simulink model "PubIfDecisionTOS_MDL"  (R2020b)
settings: configuration reference "DspaceConfig" (kept outside this file)
PostLoadFcn:
  | if any(exist('dsrtsu_mdlpostloadfcn', 'file') ~= 0), dsrtsu_mdlpostloadfcn('Execute', bdroot); end
InitFcn:
  | , if any(exist('dsmpb_private', 'file') ~= 0), dsmpb_private('dsmpb_mdlclblib', 'Init', bdroot); end,
undefined symbols (not defined in the file or in its folder): C_TOS_ACCEgoRAxletoFbumplength_m, C_TOS_ACCTargetFront_Flag, C_TOS_AEBJAPedObjDxThre_Val, C_TOS_AEBJAPedObjDyThre_Val, C_TOS_AEBJATargetSize_Val, C_TOS_AEBJAVehObjDxThre_Val, C_TOS_AEBJAVehObjDyThre_Val, C_TOS_AEBJuncPedTargetSize_Val, C_TOS_AEBLatObjDxThre_Val, C_TOS_AEBLatPedDyThre_Val, C_TOS_AEBLatTargetSize_Val, C_TOS_AEBLongTargetInEgoFront_Flag, C_TOS_axAbsGround_Parameter, C_TOS_CameraConfirmedFlag, C_TOS_CNsubjWidth, C_TOS_CurrentLaneCoreMinWidth_Val, C_TOS_CutInProb_Val_Zero, C_TOS_CutOutProb_Val_Zero, C_TOS_D2R_Val, C_TOS_DefaultValueObjectToCenterLine_dy, C_TOS_EgoCarWidth_Val, C_TOS_EgoDxRefPoint_m, C_TOS_EgoRAxletoFbumplength_m, C_TOS_HalfWidthVehicle_Con, C_TOS_HWA_CurrentLaneFlag, C_TOS_HWA_LeftLaneFlag, C_TOS_HWA_MovingDir_Vaild, C_TOS_HWA_MovState_Vaild, C_TOS_HWA_RightLaneFlag, C_TOS_LaneLineCourseErrorFront, C_TOS_LaneLineCourseErrorRear, C_TOS_MotorbikeDefaultWidth_m, C_TOS_NumberOfEffectiveTargets, C_TOS_Obj_Age_Val, C_TOS_Objdx_Constraint_Val, C_TOS_ObjectDefaultWidth_m, C_TOS_ObjInCurrentLane_Val, C_TOS_ObjInCurrentLaneValid, C_TOS_ObjInLeftLaneValid, C_TOS_ObjInRightLaneValid, C_TOS_ObjNotInCurrentLane_Val, C_TOS_ObjNotREElementType, C_TOS_ObjPredictDis_dy_ConstantVal_Zeros, C_TOS_ObjToCenterLine_ConstantVal_Zeros, C_TOS_OFMObjIDInvilad_Val, C_TOS_PIL_LatDisCons_Val_zero, C_TOS_PIL_ObjectCutInFlag_b, C_TOS_PIL_ObjectCutOutFlag_b, C_TOS_PIL_ObjLaneProb_al_Val, C_TOS_PP_ObjFusType_FC_Confirm_b, C_TOS_PP_ObjFusType_FC_FR_Confirm_b, C_TOS_PP_ObjFusType_FR_Confirm_b, C_TOS_RE_80BoolDefault_Val, C_TOS_RE_80Single181Default_Val, C_TOS_RE_80Single255Default_Val, C_TOS_RE_80Uint8Default_Val, C_TOS_RE_D2R, C_TOS_RE_D_180_Val, C_TOS_RE_InvalidObjectID_Val, C_TOS_RE_InvalidTargetChainDir_Val ... (+142)
libraries: simulink x1650, TOS_LIB x361, canfdmsglib x14
(part 50 of 69)

== system PubIfDecisionTOS_MDL/TOS_20201112/TOS_2012080320/PP1128/AAT-AdditionalAttributes/RoadEdge/RE_2020_12_07/RoadEdge_V2/RoadEdgeElementFinalJudge/EgoRight_RoadEdgeElementsFinalJudge/Dy_Filter/If Action Subsystem ==
  Object_Dy : Inport
  Action Port : ActionPort  ActionPortLabel=if(u1|u2)
  Object_DyFilter : Outport
  wires:
  Object_Dy/1 -> Object_DyFilter/1

== system PubIfDecisionTOS_MDL/TOS_20201112/TOS_2012080320/PP1128/AAT-AdditionalAttributes/RoadEdge/RE_2020_12_07/RoadEdge_V2/RoadEdgeElementFinalJudge/EgoRight_RoadEdgeElementsFinalJudge/Dy_Filter/Subsystem ==
  Object_Dy : Inport
  Object_Dy_K1 : Inport  Port=2
  Action Port : ActionPort  ActionPortLabel=else
  Abs : Abs
  Add : Sum  Inputs=+-
  Add1 : Sum
  Constant : Constant  Value=0.2  OutDataTypeStr=single
  Gain : Gain  Gain=0.5
  Relational Operator : RelationalOperator  Operator=<  OutDataTypeStr=boolean  RndMeth=Simplest
  Switch : Switch  Criteria=u2 ~= 0
  Object_DyFilter : Outport
  wires:
  Constant/1 -> Relational Operator/2
  Object_Dy/1 -> Switch/1, Add/1
  Gain/1 -> Add1/1
  Object_Dy_K1/1 -> Add1/2, Add/2
  Abs/1 -> Relational Operator/1
  Add/1 -> Gain/1, Abs/1
  Relational Operator/1 -> Switch/2
  Add1/1 -> Switch/3
  Switch/1 -> Object_DyFilter/1

== system PubIfDecisionTOS_MDL/TOS_20201112/TOS_2012080320/PP1128/AAT-AdditionalAttributes/RoadEdge/RE_2020_12_07/RoadEdge_V2/SelectStationaryObjects/SelectStationaryObject/RE_StationaryObjectsSortCond/RE_Object_DxDy ==
  Object_Dx : Inport
  Object_Dy : Inport  Port=2
  Abs : Abs
  Compare To Constant : simulink/Logic and Bit Operations/Compare To Constant  relop=<=  const=P_TOS_RE_TargetDxMaxVal_m  OutDataTypeStr=boolean
      settings: AttributesFormatString=%<const> = 200
  Compare To Constant1 : simulink/Logic and Bit Operations/Compare To Constant  relop=>=  const=P_TOS_RE_TargetDxMinVal_m  OutDataTypeStr=boolean
      settings: AttributesFormatString=%<const> = 0
  Compare To Constant2 : simulink/Logic and Bit Operations/Compare To Constant  relop=<=  const=P_TOS_RE_TargetDyMaxVal_m  OutDataTypeStr=boolean
      settings: AttributesFormatString=%<const> = 20
  Compare To Constant3 : simulink/Logic and Bit Operations/Compare To Constant  relop=>  const=P_TOS_RE_TargetDyMinVal_m  OutDataTypeStr=boolean
      settings: AttributesFormatString=%<const> = 0.5
  Logical Operator1 : Logic  AllPortsSameDT=off  OutDataTypeStr=boolean
  Logical Operator2 : Logic  AllPortsSameDT=off  OutDataTypeStr=boolean
  Logical Operator3 : Logic  AllPortsSameDT=off  OutDataTypeStr=boolean
  RE_Object_DxDy : Outport
  wires:
  Logical Operator1/1 -> RE_Object_DxDy/1
  Object_Dx/1 -> Compare To Constant1/1, Compare To Constant/1
  Compare To Constant/1 -> Logical Operator2/1
  Compare To Constant1/1 -> Logical Operator2/2
  Logical Operator2/1 -> Logical Operator1/1
  Object_Dy/1 -> Abs/1
  Abs/1 -> Compare To Constant3/1, Compare To Constant2/1
  Compare To Constant2/1 -> Logical Operator3/1
  Compare To Constant3/1 -> Logical Operator3/2
  Logical Operator3/1 -> Logical Operator1/2

== system PubIfDecisionTOS_MDL/TOS_20201112/TOS_2012080320/PP1128/AAT-AdditionalAttributes/RoadEdge/RE_2020_12_07/RoadEdge_V2/SelectStationaryObjects/SelectStationaryObject/RE_StationaryObjectsSortCond/RE_Object_DxDyStd ==
  Object_DxStd : Inport
  Object_DyStd : Inport  Port=2
  Compare To Constant : simulink/Logic and Bit Operations/Compare To Constant  relop=<=  const=P_TOS_RE_TargetDxStdMaxVal  OutDataTypeStr=boolean
      settings: AttributesFormatString=%<const> = 12.5
  Compare To Constant2 : simulink/Logic and Bit Operations/Compare To Constant  relop=<=  const=P_TOS_RE_TargetDyStdMaxVal  OutDataTypeStr=boolean
      settings: AttributesFormatString=%<const> = 12.5
  Logical Operator1 : Logic  AllPortsSameDT=off  OutDataTypeStr=boolean
  RE_Object_DxDyStd : Outport
  wires:
  Compare To Constant2/1 -> Logical Operator1/2
  Object_DyStd/1 -> Compare To Constant2/1
  Compare To Constant/1 -> Logical Operator1/1
  Object_DxStd/1 -> Compare To Constant/1
  Logical Operator1/1 -> RE_Object_DxDyStd/1

== system PubIfDecisionTOS_MDL/TOS_20201112/TOS_2012080320/PP1128/AAT-AdditionalAttributes/RoadEdge/RE_2020_12_07/RoadEdge_V2/SelectStationaryObjects/SelectStationaryObject/RE_StationaryObjectsSortCond/RE_Object_FusType ==
  Object_FusType : Inport
  Data Type Conversion : DataTypeConversion  OutDataTypeStr=Enum: OFM_OBJ_FUSTYPE
  Enumerated Constant63 : simulink/Sources/Enumerated Constant  OutDataTypeStr=Enum: OFM_OBJ_FUSTYPE  Value=OFM_OBJ_FUSTYPE.FR  SampleTime=inf
      settings: AttributesFormatString=OFM_OBJ_FUSTYPE.FR = 2
  Enumerated Constant65 : simulink/Sources/Enumerated Constant  OutDataTypeStr=Enum: OFM_OBJ_FUSTYPE  Value=OFM_OBJ_FUSTYPE.FR_CL  SampleTime=inf
      settings: AttributesFormatString=OFM_OBJ_FUSTYPE.FR_CL = 6
  Enumerated Constant67 : simulink/Sources/Enumerated Constant  OutDataTypeStr=Enum: OFM_OBJ_FUSTYPE  Value=OFM_OBJ_FUSTYPE.FR_CR  SampleTime=inf
      settings: AttributesFormatString=OFM_OBJ_FUSTYPE.FR_CR = 10
  Enumerated Constant69 : simulink/Sources/Enumerated Constant  OutDataTypeStr=Enum: OFM_OBJ_FUSTYPE  Value=OFM_OBJ_FUSTYPE.FR_CL_CR  SampleTime=inf
      settings: AttributesFormatString=OFM_OBJ_FUSTYPE.FR_CL_CR = 14
  Enumerated Constant71 : simulink/Sources/Enumerated Constant  OutDataTypeStr=Enum: OFM_OBJ_FUSTYPE  Value=OFM_OBJ_FUSTYPE.FR_BL  SampleTime=inf
      settings: AttributesFormatString=OFM_OBJ_FUSTYPE.FR_BL = 18
  Enumerated Constant73 : simulink/Sources/Enumerated Constant  OutDataTypeStr=Enum: OFM_OBJ_FUSTYPE  Value=OFM_OBJ_FUSTYPE.FR_CL_BL  SampleTime=inf
      settings: AttributesFormatString=OFM_OBJ_FUSTYPE.FR_CL_BL = 22
  Enumerated Constant75 : simulink/Sources/Enumerated Constant  OutDataTypeStr=Enum: OFM_OBJ_FUSTYPE  Value=OFM_OBJ_FUSTYPE.FR_CR_BL  SampleTime=inf
      settings: AttributesFormatString=OFM_OBJ_FUSTYPE.FR_CR_BL = 26
  Enumerated Constant77 : simulink/Sources/Enumerated Constant  OutDataTypeStr=Enum: OFM_OBJ_FUSTYPE  Value=OFM_OBJ_FUSTYPE.FR_CL_CR_BL  SampleTime=inf
      settings: AttributesFormatString=OFM_OBJ_FUSTYPE.FR_CL_CR_BL = 30
  Enumerated Constant79 : simulink/Sources/Enumerated Constant  OutDataTypeStr=Enum: OFM_OBJ_FUSTYPE  Value=OFM_OBJ_FUSTYPE.FR_BR  SampleTime=inf
      settings: AttributesFormatString=OFM_OBJ_FUSTYPE.FR_BR = 34
  Enumerated Constant81 : simulink/Sources/Enumerated Constant  OutDataTypeStr=Enum: OFM_OBJ_FUSTYPE  Value=OFM_OBJ_FUSTYPE.FR_CL_BR  SampleTime=inf
      settings: AttributesFormatString=OFM_OBJ_FUSTYPE.FR_CL_BR = 38
  Enumerated Constant83 : simulink/Sources/Enumerated Constant  OutDataTypeStr=Enum: OFM_OBJ_FUSTYPE  Value=OFM_OBJ_FUSTYPE.FR_CR_BR  SampleTime=inf
      settings: AttributesFormatString=OFM_OBJ_FUSTYPE.FR_CR_BR = 42
  Enumerated Constant85 : simulink/Sources/Enumerated Constant  OutDataTypeStr=Enum: OFM_OBJ_FUSTYPE  Value=OFM_OBJ_FUSTYPE.FR_CL_CR_BR  SampleTime=inf
      settings: AttributesFormatString=OFM_OBJ_FUSTYPE.FR_CL_CR_BR = 46
  Enumerated Constant87 : simulink/Sources/Enumerated Constant  OutDataTypeStr=Enum: OFM_OBJ_FUSTYPE  Value=OFM_OBJ_FUSTYPE.FR_BL_BR  SampleTime=inf
      settings: AttributesFormatString=OFM_OBJ_FUSTYPE.FR_BL_BR = 50
  Enumerated Constant89 : simulink/Sources/Enumerated Constant  OutDataTypeStr=Enum: OFM_OBJ_FUSTYPE  Value=OFM_OBJ_FUSTYPE.FR_CL_BL_BR  SampleTime=inf
      settings: AttributesFormatString=OFM_OBJ_FUSTYPE.FR_CL_BL_BR = 54
  Enumerated Constant91 : simulink/Sources/Enumerated Constant  OutDataTypeStr=Enum: OFM_OBJ_FUSTYPE  Value=OFM_OBJ_FUSTYPE.FR_CR_BL_BR  SampleTime=inf
      settings: AttributesFormatString=OFM_OBJ_FUSTYPE.FR_CR_BL_BR = 58
  Enumerated Constant93 : simulink/Sources/Enumerated Constant  OutDataTypeStr=Enum: OFM_OBJ_FUSTYPE  Value=OFM_OBJ_FUSTYPE.FR_CL_CR_BL_BR  SampleTime=inf
      settings: AttributesFormatString=OFM_OBJ_FUSTYPE.FR_CL_CR_BL_BR = 62
  Logical Operator15 : Logic  Operator=OR  Inputs=16  AllPortsSameDT=off  OutDataTypeStr=boolean
  Relational Operator{16,20,22,24,26,28,30,32,34,36,38,40,42,44,46,48} (16 alike) : RelationalOperator  Operator===  OutDataTypeStr=boolean  RndMeth=Nearest
  RE_Object_FR_Other : Outport
  wires:
  Logical Operator15/1 -> RE_Object_FR_Other/1
  Enumerated Constant63/1 -> Relational Operator16/2
  Enumerated Constant65/1 -> Relational Operator20/2
  Enumerated Constant69/1 -> Relational Operator24/2
  Enumerated Constant67/1 -> Relational Operator22/2
  Enumerated Constant75/1 -> Relational Operator30/2
  Enumerated Constant77/1 -> Relational Operator32/2
  Enumerated Constant73/1 -> Relational Operator28/2
  Enumerated Constant71/1 -> Relational Operator26/2
  Enumerated Constant87/1 -> Relational Operator42/2
  Enumerated Constant89/1 -> Relational Operator44/2
  Enumerated Constant93/1 -> Relational Operator48/2
  Enumerated Constant91/1 -> Relational Operator46/2
  Object_FusType/1 -> Data Type Conversion/1
  Enumerated Constant83/1 -> Relational Operator38/2
  Enumerated Constant85/1 -> Relational Operator40/2
  Enumerated Constant81/1 -> Relational Operator36/2
  Enumerated Constant79/1 -> Relational Operator34/2
  Relational Operator16/1 -> Logical Operator15/1
  Relational Operator48/1 -> Logical Operator15/16
  Data Type Conversion/1 -> Relational Operator20/1, Relational Operator22/1, Relational Operator24/1, Relational Operator26/1, Relational Operator28/1, Relational Operator30/1, Relational Operator32/1, Relational Operator34/1, Relational Operator36/1, Relational Operator38/1, Relational Operator40/1, Relational Operator42/1, Relational Operator44/1, Relational Operator46/1, Relational Operator48/1, Relational Operator16/1
  Relational Operator20/1 -> Logical Operator15/2
  Relational Operator22/1 -> Logical Operator15/3
  Relational Operator24/1 -> Logical Operator15/4
  Relational Operator26/1 -> Logical Operator15/5
  Relational Operator28/1 -> Logical Operator15/6
  Relational Operator30/1 -> Logical Operator15/7
  Relational Operator32/1 -> Logical Operator15/8
  Relational Operator34/1 -> Logical Operator15/9
  Relational Operator36/1 -> Logical Operator15/10
  Relational Operator38/1 -> Logical Operator15/11
  Relational Operator40/1 -> Logical Operator15/12
  Relational Operator42/1 -> Logical Operator15/13
  Relational Operator44/1 -> Logical Operator15/14
  Relational Operator46/1 -> Logical Operator15/15

== system PubIfDecisionTOS_MDL/TOS_20201112/TOS_2012080320/PP1128/AAT-AdditionalAttributes/RoadEdge/RE_2020_12_07/RoadEdge_V2/SelectStationaryObjects/SelectStationaryObject/RE_StationaryObjectsSortCond/RE_Object_MovingState ==
  Object_MovingState : Inport
  Compare To Constant : simulink/Logic and Bit Operations/Compare To Constant  relop===  const=OFM_OBJ_MOVINGSTATE_E.STATIONARY  OutDataTypeStr=boolean
      settings: AttributesFormatString=%<const>
  Data Type Conversion1 : DataTypeConversion  OutDataTypeStr=Enum: OFM_OBJ_MOVINGSTATE_E
  RE_Object_Stationary : Outport
  wires:
  Data Type Conversion1/1 -> Compare To Constant/1
  Object_MovingState/1 -> Data Type Conversion1/1
  Compare To Constant/1 -> RE_Object_Stationary/1

== system PubIfDecisionTOS_MDL/TOS_20201112/TOS_2012080320/PP1128/AAT-AdditionalAttributes/RoadEdge/RE_2020_12_07/RoadEdge_V2/SelectStationaryObjects/SelectStationaryObject/RE_StationaryObjectsSortCond/Subsystem ==
  Object_ExistProb : Inport
  Object_ExistProb_K1 : Inport  Port=2
  Compare To Constant : simulink/Logic and Bit Operations/Compare To Constant  relop=>=  const=P_TOS_RE_ExistProbThre_val  OutDataTypeStr=boolean
      settings: AttributesFormatString="%<const>  = 0.4"
  Compare To Constant1 : simulink/Logic and Bit Operations/Compare To Constant  relop=>=  const=P_TOS_RE_ExistProbThre_val  OutDataTypeStr=boolean
      settings: AttributesFormatString="%<const>  = 0.4"
  Constant : Constant  Value=P_TOS_RE_stateProlongationTime  OutDataTypeStr=single
      settings: AttributesFormatString=%<Value> = 0.2
  Constant1 : Constant  Value=P_TOS_RE_Ts  OutDataTypeStr=single
      settings: AttributesFormatString=%<Value> = 0.05
  StateDelayAbortion : Stateflow chart  TreatAsAtomicUnit=on
  Terminator : Terminator
  RE_Object_ExistProb : Outport
  wires:
  Object_ExistProb/1 -> Compare To Constant/1
  Compare To Constant/1 -> StateDelayAbortion/1(state)
  StateDelayAbortion/2(stateOut) -> RE_Object_ExistProb/1
  StateDelayAbortion/1(timeSinceLastState) -> Terminator/1
  Object_ExistProb_K1/1 -> Compare To Constant1/1
  Compare To Constant1/1 -> StateDelayAbortion/2(stateK1)
  Constant/1 -> StateDelayAbortion/3(stateProlongationTime)
  Constant1/1 -> StateDelayAbortion/4(Ts)

== system PubIfDecisionTOS_MDL/TOS_20201112/TOS_2012080320/PP1128/AAT-AdditionalAttributes/RoadEdge/RE_2020_12_07/RoadEdge_V2/TargetChain/EgoLeftTargetChainDirection/Dy_Filter/If Action Subsystem ==
  Object_Dy : Inport
  Action Port : ActionPort  ActionPortLabel=if(u1|u2)
  Object_DyFilter : Outport
  wires:
  Object_Dy/1 -> Object_DyFilter/1

== system PubIfDecisionTOS_MDL/TOS_20201112/TOS_2012080320/PP1128/AAT-AdditionalAttributes/RoadEdge/RE_2020_12_07/RoadEdge_V2/TargetChain/EgoLeftTargetChainDirection/Dy_Filter/Subsystem ==
  Object_Dy : Inport
  Object_Dy_K1 : Inport  Port=2
  Action Port : ActionPort  ActionPortLabel=else
  Abs : Abs
  Add : Sum  Inputs=+-
  Add1 : Sum
  Constant : Constant  Value=0.2  OutDataTypeStr=single
  Gain : Gain  Gain=0.5
  Relational Operator : RelationalOperator  Operator=<  OutDataTypeStr=boolean  RndMeth=Simplest
  Switch : Switch  Criteria=u2 ~= 0
  Object_DyFilter : Outport
  wires:
  Constant/1 -> Relational Operator/2
  Object_Dy/1 -> Switch/1, Add/1
  Gain/1 -> Add1/1
  Object_Dy_K1/1 -> Add1/2, Add/2
  Abs/1 -> Relational Operator/1
  Add/1 -> Gain/1, Abs/1
  Relational Operator/1 -> Switch/2
  Add1/1 -> Switch/3
  Switch/1 -> Object_DyFilter/1

== system PubIfDecisionTOS_MDL/TOS_20201112/TOS_2012080320/PP1128/AAT-AdditionalAttributes/RoadEdge/RE_2020_12_07/RoadEdge_V2/TargetChain/EgoRightTargetChainDirection/Dy_Filter/If Action Subsystem ==
  Object_Dy : Inport
  Action Port : ActionPort  ActionPortLabel=if(u1|u2)
  Object_DyFilter : Outport
  wires:
  Object_Dy/1 -> Object_DyFilter/1

== system PubIfDecisionTOS_MDL/TOS_20201112/TOS_2012080320/PP1128/AAT-AdditionalAttributes/RoadEdge/RE_2020_12_07/RoadEdge_V2/TargetChain/EgoRightTargetChainDirection/Dy_Filter/Subsystem ==
  Object_Dy : Inport
  Object_Dy_K1 : Inport  Port=2
  Action Port : ActionPort  ActionPortLabel=else
  Abs : Abs
  Add : Sum  Inputs=+-
  Add1 : Sum
  Constant : Constant  Value=0.2  OutDataTypeStr=single
  Gain : Gain  Gain=0.5
  Relational Operator : RelationalOperator  Operator=<  OutDataTypeStr=boolean  RndMeth=Simplest
  Switch : Switch  Criteria=u2 ~= 0
  Object_DyFilter : Outport
  wires:
  Constant/1 -> Relational Operator/2
  Object_Dy/1 -> Switch/1, Add/1
  Gain/1 -> Add1/1
  Object_Dy_K1/1 -> Add1/2, Add/2
  Abs/1 -> Relational Operator/1
  Add/1 -> Gain/1, Abs/1
  Relational Operator/1 -> Switch/2
  Add1/1 -> Switch/3
  Switch/1 -> Object_DyFilter/1

== system PubIfDecisionTOS_MDL/TOS_20201112/TOS_2012080320/TOS/ACC/TOS_ACCCurrentLane/ACC_CurrentLane_Target/TOS_ACC_P0/ACC_P0_Targe/ACC_P0_Targe/TOS_ACC_DyConfirm/OverLapConfirm ==
  note: 弯道小于1000m,使用overlap
  note: R = 1200m
  DyConfirm_Sig : Inport
  Abs{,1..3} (4 alike) : Abs
  Add : Sum
  Bus Creator{1..4} (4 alike) : BusCreator  Inputs=2
  Bus Selector : BusSelector  OutputSignals=PositionFlag,Line_pC2
  Bus Selector1 : BusSelector  OutputSignals=PositionFlag,Line_pC2
  Bus Selector2 : BusSelector  OutputSignals=LM_LR_Line04_pC0,LM_RL_Line04_pC0
  Bus Selector3 : BusSelector  OutputSignals=PositionFlag,Line_pC2
  Bus Selector4 : BusSelector  OutputSignals=LM_LR_Line04_pC2,Object_DX,LM_LR_Line04_dDisStart,LM_LR_Line04_dDisEnd,LM_LR_Line04_fCamValid
  Bus Selector5 : BusSelector  OutputSignals=LM_LR_Line05_pC2,Object_DX,LM_LR_Line05_dDisStart,LM_LR_Line05_dDisEnd,LM_LR_Line05_fCamValid
  Bus Selector8 : BusSelector  OutputSignals=LM_LR_Line06_pC2,Object_DX,LM_LR_Line06_dDisStart,LM_LR_Line06_dDisEnd,LM_LR_Line06_fCamValid
  Compare To Constant : simulink/Logic and Bit Operations/Compare To Constant  relop===  const=uint8(4)  OutDataTypeStr=boolean
  Compare To Constant1 : simulink/Logic and Bit Operations/Compare To Constant  relop=>=  const=single(0.001)  OutDataTypeStr=boolean
  Compare To Constant2 : simulink/Logic and Bit Operations/Compare To Constant  relop=<=  const=single(0.1)  OutDataTypeStr=boolean
  Compare To Constant3 : simulink/Logic and Bit Operations/Compare To Constant  relop===  const=uint8(5)  OutDataTypeStr=boolean
  Compare To Constant4 : simulink/Logic and Bit Operations/Compare To Constant  relop=>=  const=single(0.001)  OutDataTypeStr=boolean
  Compare To Constant5 : simulink/Logic and Bit Operations/Compare To Constant  relop===  const=uint8(6)  OutDataTypeStr=boolean
  Compare To Constant6 : simulink/Logic and Bit Operations/Compare To Constant  relop=>=  const=single(0.001)  OutDataTypeStr=boolean
  Constant : Constant  Value=0  OutDataTypeStr=uint8
  Constant1 : Constant  Value=4  OutDataTypeStr=uint8
  Constant2 : Constant  Value=5  OutDataTypeStr=uint8
  Constant3 : Constant  Value=6  OutDataTypeStr=uint8
  Constant4 : Constant  Value=0  OutDataTypeStr=single
  Constant5 : Constant  OutDataTypeStr=boolean
  Logical Operator1 : Logic  AllPortsSameDT=off  OutDataTypeStr=boolean
  Logical Operator10 : Logic  Inputs=3  AllPortsSameDT=off  OutDataTypeStr=boolean
  Logical Operator11 : Logic  Inputs=3  AllPortsSameDT=off  OutDataTypeStr=boolean
  Logical Operator2 : Logic  AllPortsSameDT=off  OutDataTypeStr=boolean
  Logical Operator3 : Logic  AllPortsSameDT=off  OutDataTypeStr=boolean
  Logical Operator4 : Logic  Operator=OR  Inputs=3  AllPortsSameDT=off  OutDataTypeStr=boolean
  Logical Operator5 : Logic  Operator=OR  AllPortsSameDT=off  OutDataTypeStr=boolean
  Logical Operator6 : Logic  Operator=OR  AllPortsSameDT=off  OutDataTypeStr=boolean
  Logical Operator7 : Logic  Operator=OR  AllPortsSameDT=off  OutDataTypeStr=boolean
  Logical Operator9 : Logic  Inputs=3  AllPortsSameDT=off  OutDataTypeStr=boolean
  Relational Operator4 : RelationalOperator  Operator=>  OutDataTypeStr=boolean  RndMeth=Simplest
  Relational Operator5 : RelationalOperator  Operator=<=  OutDataTypeStr=boolean  RndMeth=Simplest
  Relational Operator6 : RelationalOperator  Operator=>  OutDataTypeStr=boolean  RndMeth=Simplest
  Relational Operator7 : RelationalOperator  Operator=<=  OutDataTypeStr=boolean  RndMeth=Simplest
  Relational Operator8 : RelationalOperator  Operator=>  OutDataTypeStr=boolean  RndMeth=Simplest
  Relational Operator9 : RelationalOperator  Operator=<=  OutDataTypeStr=boolean  RndMeth=Simplest
  Signal Copy : SignalConversion  OverrideOpt=off
  Signal Copy1 : SignalConversion  OverrideOpt=off
  Signal Copy2 : SignalConversion  OverrideOpt=off
  Switch3 : Switch  Criteria=u2 > Threshold  OutDataTypeStr=single
  Switch4 : Switch  Criteria=u2 > Threshold  OutDataTypeStr=single
  Switch5 : Switch  Criteria=u2 > Threshold  OutDataTypeStr=single
  Terminator : Terminator
  TOS_ACC_OverlapRatio : Outport
  wires:
  Abs3/1 -> Compare To Constant2/1
  Add/1 -> Abs3/1
  Logical Operator7/1 -> Logical Operator11/3
  [C0_Confirm] -> Logical Operator7/2
  Logical Operator6/1 -> Logical Operator10/3
  [C0_Confirm] -> Logical Operator6/2
  Logical Operator5/1 -> Logical Operator9/3
  [C0_Confirm] -> Logical Operator5/2
  Compare To Constant2/1 -> Terminator/1
  Bus Selector2/2 -> Add/2  "<LM_RL_Line04_pC0>"
  Bus Selector2/1 -> Add/1  "<LM_LR_Line04_pC0>"
  Abs2/1 -> Compare To Constant6/1
  Abs1/1 -> Compare To Constant4/1
  Abs/1 -> Compare To Constant1/1
  Logical Operator4/1 -> TOS_ACC_OverlapRatio/1
  Logical Operator3/1 -> Logical Operator4/3
  Logical Operator2/1 -> Logical Operator4/2
  Bus Selector3/2 -> Abs2/1  "<Line_pC2>"
  Bus Selector3/1 -> Compare To Constant5/1  "<PositionFlag>"
  Switch3/1 -> Bus Selector/1, Bus Selector1/1, Bus Selector3/1
  Compare To Constant5/1 -> Logical Operator3/1
  Compare To Constant6/1 -> Logical Operator3/2
  Compare To Constant4/1 -> Logical Operator2/2
  Compare To Constant3/1 -> Logical Operator2/1
  Bus Selector1/1 -> Compare To Constant3/1  "<PositionFlag>"
  Bus Selector1/2 -> Abs1/1  "<Line_pC2>"
  Logical Operator1/1 -> Logical Operator4/1
  Compare To Constant1/1 -> Logical Operator1/2
  DyConfirm_Sig/1 -> Bus Selector2/1, Bus Selector4/1, Bus Selector5/1, Bus Selector8/1
  Compare To Constant/1 -> Logical Operator1/1
  Bus Selector/2 -> Abs/1  "<Line_pC2>"
  Bus Selector/1 -> Compare To Constant/1  "<PositionFlag>"
  Constant4/1 -> Bus Creator4/2  "Line_pC2"
  Bus Creator3/1 -> Switch5/1
  Signal Copy2/1 -> Bus Creator3/2  "Line_pC2"
  Bus Selector4/1 -> Signal Copy/1  "<LM_LR_Line04_pC2>"
  Logical Operator9/1 -> Switch3/2
  Bus Selector5/1 -> Signal Copy1/1  "<LM_LR_Line05_pC2>"
  Constant/1 -> Bus Creator4/1  "PositionFlag"
  Signal Copy1/1 -> Bus Creator2/2  "Line_pC2"
  Constant3/1 -> Bus Creator3/1  "PositionFlag"
  Constant2/1 -> Bus Creator2/1  "PositionFlag"
  Bus Selector4/4 -> Relational Operator5/2  "<LM_LR_Line04_dDisEnd>"
  Bus Creator4/1 -> Switch5/3
  Relational Operator7/1 -> Logical Operator10/2
  Relational Operator6/1 -> Logical Operator10/1
  Constant1/1 -> Bus Creator1/1  "PositionFlag"
  Relational Operator4/1 -> Logical Operator9/1
  Bus Creator2/1 -> Switch4/1
  Bus Selector5/5 -> Logical Operator6/1  "<LM_LR_Line05_fCamValid>"
  Switch5/1 -> Switch4/3
  Bus Selector8/5 -> Logical Operator7/1  "<LM_LR_Line06_fCamValid>"
  Bus Selector5/2 -> Relational Operator7/1, Relational Operator6/1  "<Object_DX>"
  Bus Selector5/3 -> Relational Operator6/2  "<LM_LR_Line05_dDisStart>"
  Logical Operator11/1 -> Switch5/2
  Bus Creator1/1 -> Switch3/1
  Bus Selector8/4 -> Relational Operator9/2  "<LM_LR_Line06_dDisEnd>"
  Switch4/1 -> Switch3/3
  Relational Operator9/1 -> Logical Operator11/2
  Bus Selector8/1 -> Signal Copy2/1  "<LM_LR_Line06_pC2>"
  Bus Selector8/3 -> Relational Operator8/2  "<LM_LR_Line06_dDisStart>"
  Signal Copy/1 -> Bus Creator1/2  "Line_pC2"
  Relational Operator5/1 -> Logical Operator9/2
  Relational Operator8/1 -> Logical Operator11/1
  Bus Selector4/2 -> Relational Operator4/1, Relational Operator5/1  "<Object_DX>"
  Bus Selector5/4 -> Relational Operator7/2  "<LM_LR_Line05_dDisEnd>"
  Bus Selector4/3 -> Relational Operator4/2  "<LM_LR_Line04_dDisStart>"
  Bus Selector4/5 -> Logical Operator5/1  "<LM_LR_Line04_fCamValid>"
  Bus Selector8/2 -> Relational Operator8/1, Relational Operator9/1  "<Object_DX>"
  Logical Operator10/1 -> Switch4/2
  Constant5/1 -> [C0_Confirm]

== system PubIfDecisionTOS_MDL/TOS_20201112/TOS_2012080320/TOS/ACC/TOS_ACCCurrentLane/ACC_CurrentLane_Target/TOS_ACC_P0/ACC_P0_Targe/ACC_P0_Targe/TOS_ACC_DyConfirm/OverLapConfirm_V0318（） ==
  note: R = 1200m
  DyConfirm_Sig : Inport
  Abs{,1..3} (4 alike) : Abs
  Add : Sum
  Bus Creator{1..4} (4 alike) : BusCreator  Inputs=2
  Bus Selector : BusSelector  OutputSignals=PositionFlag,Line_pC2
  Bus Selector1 : BusSelector  OutputSignals=PositionFlag,Line_pC2
  Bus Selector2 : BusSelector  OutputSignals=LM_LR_Line04_pC0,LM_RL_Line04_pC0
  Bus Selector3 : BusSelector  OutputSignals=PositionFlag,Line_pC2
  Bus Selector4 : BusSelector  OutputSignals=LM_LR_Line04_pC2,Object_DX,LM_LR_Line04_dDisStart,LM_LR_Line04_dDisEnd,LM_LR_Line04_fCamValid
  Bus Selector5 : BusSelector  OutputSignals=LM_LR_Line05_pC2,Object_DX,LM_LR_Line05_dDisStart,LM_LR_Line05_dDisEnd,LM_LR_Line05_fCamValid
  Bus Selector8 : BusSelector  OutputSignals=LM_LR_Line06_pC2,Object_DX,LM_LR_Line06_dDisStart,LM_LR_Line06_dDisEnd,LM_LR_Line06_fCamValid
  Compare To Constant : simulink/Logic and Bit Operations/Compare To Constant  relop===  const=uint8(4)  OutDataTypeStr=boolean
  Compare To Constant1 : simulink/Logic and Bit Operations/Compare To Constant  relop=>=  const=single(0.001)  OutDataTypeStr=boolean
  Compare To Constant2 : simulink/Logic and Bit Operations/Compare To Constant  relop=<=  const=single(0.1)  OutDataTypeStr=boolean
  Compare To Constant3 : simulink/Logic and Bit Operations/Compare To Constant  relop===  const=uint8(5)  OutDataTypeStr=boolean
  Compare To Constant4 : simulink/Logic and Bit Operations/Compare To Constant  relop=>=  const=single(0.001)  OutDataTypeStr=boolean
  Compare To Constant5 : simulink/Logic and Bit Operations/Compare To Constant  relop===  const=uint8(6)  OutDataTypeStr=boolean
  Compare To Constant6 : simulink/Logic and Bit Operations/Compare To Constant  relop=>=  const=single(0.001)  OutDataTypeStr=boolean
  Constant : Constant  Value=0  OutDataTypeStr=uint8
  Constant1 : Constant  Value=4  OutDataTypeStr=uint8
  Constant2 : Constant  Value=5  OutDataTypeStr=uint8
  Constant3 : Constant  Value=6  OutDataTypeStr=uint8
  Constant4 : Constant  Value=0  OutDataTypeStr=single
  Logical Operator1 : Logic  AllPortsSameDT=off  OutDataTypeStr=boolean
  Logical Operator10 : Logic  Inputs=3  AllPortsSameDT=off  OutDataTypeStr=boolean
  Logical Operator11 : Logic  Inputs=3  AllPortsSameDT=off  OutDataTypeStr=boolean
  Logical Operator2 : Logic  AllPortsSameDT=off  OutDataTypeStr=boolean
  Logical Operator3 : Logic  AllPortsSameDT=off  OutDataTypeStr=boolean
  Logical Operator4 : Logic  Operator=OR  Inputs=3  AllPortsSameDT=off  OutDataTypeStr=boolean
  Logical Operator5 : Logic  Operator=OR  AllPortsSameDT=off  OutDataTypeStr=boolean
  Logical Operator6 : Logic  Operator=OR  AllPortsSameDT=off  OutDataTypeStr=boolean
  Logical Operator7 : Logic  Operator=OR  AllPortsSameDT=off  OutDataTypeStr=boolean
  Logical Operator9 : Logic  Inputs=3  AllPortsSameDT=off  OutDataTypeStr=boolean
  Relational Operator4 : RelationalOperator  Operator=>  OutDataTypeStr=boolean  RndMeth=Simplest
  Relational Operator5 : RelationalOperator  Operator=<=  OutDataTypeStr=boolean  RndMeth=Simplest
  Relational Operator6 : RelationalOperator  Operator=>  OutDataTypeStr=boolean  RndMeth=Simplest
  Relational Operator7 : RelationalOperator  Operator=<=  OutDataTypeStr=boolean  RndMeth=Simplest
  Relational Operator8 : RelationalOperator  Operator=>  OutDataTypeStr=boolean  RndMeth=Simplest
  Relational Operator9 : RelationalOperator  Operator=<=  OutDataTypeStr=boolean  RndMeth=Simplest
  Signal Copy : SignalConversion  OverrideOpt=off
  Signal Copy1 : SignalConversion  OverrideOpt=off
  Signal Copy2 : SignalConversion  OverrideOpt=off
  Switch3 : Switch  Criteria=u2 > Threshold  OutDataTypeStr=single
  Switch4 : Switch  Criteria=u2 > Threshold  OutDataTypeStr=single
  Switch5 : Switch  Criteria=u2 > Threshold  OutDataTypeStr=single
  TOS_ACC_OverlapRatio : Outport
  wires:
  Logical Operator10/1 -> Switch4/2
  Bus Selector8/2 -> Relational Operator9/1, Relational Operator8/1  "<Object_DX>"
  Bus Selector4/5 -> Logical Operator5/1  "<LM_LR_Line04_fCamValid>"
  Bus Selector4/3 -> Relational Operator4/2  "<LM_LR_Line04_dDisStart>"
  Bus Selector5/4 -> Relational Operator7/2  "<LM_LR_Line05_dDisEnd>"
  Bus Selector4/2 -> Relational Operator5/1, Relational Operator4/1  "<Object_DX>"
  Relational Operator8/1 -> Logical Operator11/1
  Relational Operator5/1 -> Logical Operator9/2
  Signal Copy/1 -> Bus Creator1/2  "Line_pC2"
  Bus Selector8/3 -> Relational Operator8/2  "<LM_LR_Line06_dDisStart>"
  Bus Selector8/1 -> Signal Copy2/1  "<LM_LR_Line06_pC2>"
  Relational Operator9/1 -> Logical Operator11/2
  Switch4/1 -> Switch3/3
  Bus Selector8/4 -> Relational Operator9/2  "<LM_LR_Line06_dDisEnd>"
  Bus Creator1/1 -> Switch3/1
  Logical Operator11/1 -> Switch5/2
  Bus Selector5/3 -> Relational Operator6/2  "<LM_LR_Line05_dDisStart>"
  Bus Selector5/2 -> Relational Operator6/1, Relational Operator7/1  "<Object_DX>"
  Bus Selector8/5 -> Logical Operator7/1  "<LM_LR_Line06_fCamValid>"
  Switch5/1 -> Switch4/3
  Bus Selector5/5 -> Logical Operator6/1  "<LM_LR_Line05_fCamValid>"
  Bus Creator2/1 -> Switch4/1
  Relational Operator4/1 -> Logical Operator9/1
  Constant1/1 -> Bus Creator1/1  "PositionFlag"
  Relational Operator6/1 -> Logical Operator10/1
  Relational Operator7/1 -> Logical Operator10/2
  Bus Creator4/1 -> Switch5/3
  Bus Selector4/4 -> Relational Operator5/2  "<LM_LR_Line04_dDisEnd>"
  Constant2/1 -> Bus Creator2/1  "PositionFlag"
  Constant3/1 -> Bus Creator3/1  "PositionFlag"
  Signal Copy1/1 -> Bus Creator2/2  "Line_pC2"
  Constant/1 -> Bus Creator4/1  "PositionFlag"
  Bus Selector5/1 -> Signal Copy1/1  "<LM_LR_Line05_pC2>"
  Logical Operator9/1 -> Switch3/2
  Bus Selector4/1 -> Signal Copy/1  "<LM_LR_Line04_pC2>"
  Signal Copy2/1 -> Bus Creator3/2  "Line_pC2"
  Bus Creator3/1 -> Switch5/1
  Constant4/1 -> Bus Creator4/2  "Line_pC2"
  Bus Selector/1 -> Compare To Constant/1  "<PositionFlag>"
  Bus Selector/2 -> Abs/1  "<Line_pC2>"
  Compare To Constant/1 -> Logical Operator1/1
  DyConfirm_Sig/1 -> Bus Selector8/1, Bus Selector5/1, Bus Selector4/1, Bus Selector2/1
  Compare To Constant1/1 -> Logical Operator1/2
  Logical Operator1/1 -> Logical Operator4/1
  Bus Selector1/2 -> Abs1/1  "<Line_pC2>"
  Bus Selector1/1 -> Compare To Constant3/1  "<PositionFlag>"
  Compare To Constant3/1 -> Logical Operator2/1
  Compare To Constant4/1 -> Logical Operator2/2
  Compare To Constant6/1 -> Logical Operator3/2
  Compare To Constant5/1 -> Logical Operator3/1
  Switch3/1 -> Bus Selector3/1, Bus Selector1/1, Bus Selector/1
  Bus Selector3/1 -> Compare To Constant5/1  "<PositionFlag>"
  Bus Selector3/2 -> Abs2/1  "<Line_pC2>"
  Logical Operator2/1 -> Logical Operator4/2
  Logical Operator3/1 -> Logical Operator4/3
  Logical Operator4/1 -> TOS_ACC_OverlapRatio/1
  Abs/1 -> Compare To Constant1/1
  Abs1/1 -> Compare To Constant4/1
  Abs2/1 -> Compare To Constant6/1
  Bus Selector2/1 -> Add/1  "<LM_LR_Line04_pC0>"
  Bus Selector2/2 -> Add/2  "<LM_RL_Line04_pC0>"
  Compare To Constant2/1 -> [C0_Confirm]
  [C0_Confirm] -> Logical Operator5/2
  Logical Operator5/1 -> Logical Operator9/3
  [C0_Confirm] -> Logical Operator6/2
  Logical Operator6/1 -> Logical Operator10/3
  [C0_Confirm] -> Logical Operator7/2
  Logical Operator7/1 -> Logical Operator11/3
  Add/1 -> Abs3/1
  Abs3/1 -> Compare To Constant2/1

== system PubIfDecisionTOS_MDL/TOS_20201112/TOS_2012080320/TOS/ACC/TOS_ACCCurrentLane/ACC_CurrentLane_Target/TOS_ACC_P0/ACC_P0_Targe/ACC_P0_Targe/TOS_ACC_DyConfirm/TOS_ACC_DyConfirm_V3.14 ==
  Object_DY : Inport
  Object_DX : Inport  Port=2
  <Object_Type> : Inport  Port=3
  Abs{,1..3} (4 alike) : Abs
  Bus Creator : BusCreator  Inputs=3
  Bus Selector : BusSelector  OutputSignals=Object_Type
  Bus Selector1 : BusSelector  OutputSignals=Object_DY
  Bus Selector2 : BusSelector  OutputSignals=Object_DX
  Bus Selector3 : BusSelector  OutputSignals=Object_Type
  Bus Selector4 : BusSelector  OutputSignals=Object_DY
  Bus Selector5 : BusSelector  OutputSignals=Object_DX
  Compare To Constant1 : simulink/Logic and Bit Operations/Compare To Constant  relop===  const=OFM_OBJ_TYPE_E.UNKNOWN_TYPE  OutDataTypeStr=boolean
      settings: AttributesFormatString=OFM_OBJ_TYPE_E.UNKNOWN_TYPE = 1
  Compare To Constant10 : simulink/Logic and Bit Operations/Compare To Constant  relop===  const=OFM_OBJ_TYPE_E.CAR  OutDataTypeStr=boolean
      settings: AttributesFormatString=OFM_OBJ_TYPE_E.CAR = 2
  Compare To Constant2 : simulink/Logic and Bit Operations/Compare To Constant  relop===  const=OFM_OBJ_TYPE_E.MOTORBIKE  OutDataTypeStr=boolean
      settings: AttributesFormatString=OFM_OBJ_TYPE_E.MOTORBIKE = 4
  Compare To Constant3 : simulink/Logic and Bit Operations/Compare To Constant  relop===  const=OFM_OBJ_TYPE_E.PEDESTRIAN  OutDataTypeStr=boolean
      settings: AttributesFormatString=OFM_OBJ_TYPE_E.PEDESTRIAN = 6
  Compare To Constant4 : simulink/Logic and Bit Operations/Compare To Constant  relop===  const=OFM_OBJ_TYPE_E.BICYCLE  OutDataTypeStr=boolean
      settings: AttributesFormatString=OFM_OBJ_TYPE_E.BICYCLE = 5
  Compare To Constant5 : simulink/Logic and Bit Operations/Compare To Constant  relop===  const=OFM_OBJ_TYPE_E.GENERAL_OBJECT  OutDataTypeStr=boolean
      settings: AttributesFormatString=OFM_OBJ_TYPE_E.GENERAL_OBJECT = 7
  Compare To Constant6 : simulink/Logic and Bit Operations/Compare To Constant  relop===  const=OFM_OBJ_TYPE_E.ANIMAL  OutDataTypeStr=boolean
      settings: AttributesFormatString=OFM_OBJ_TYPE_E.ANIMAL = 8
  Compare To Constant7 : simulink/Logic and Bit Operations/Compare To Constant  relop===  const=OFM_OBJ_TYPE_E.INVALID  OutDataTypeStr=boolean
      settings: AttributesFormatString=OFM_OBJ_TYPE_E.INVALID = 0
  Compare To Constant8 : simulink/Logic and Bit Operations/Compare To Constant  relop===  const=OFM_OBJ_TYPE_E.TRUCK  OutDataTypeStr=boolean
      settings: AttributesFormatString=OFM_OBJ_TYPE_E.TRUCK = 3
  Data Type Conversion1 : DataTypeConversion  OutDataTypeStr=Enum: OFM_OBJ_TYPE_E
  Data Type Conversion2 : DataTypeConversion  OutDataTypeStr=Enum: OFM_OBJ_TYPE_E
  Logical Operator : Logic  AllPortsSameDT=off  OutDataTypeStr=boolean
  Logical Operator1 : Logic  Operator=OR  Inputs=7  AllPortsSameDT=off  OutDataTypeStr=boolean
  Logical Operator2 : Logic  AllPortsSameDT=off  OutDataTypeStr=boolean
  Logical Operator3 : Logic  Operator=OR  AllPortsSameDT=off  OutDataTypeStr=boolean
  Logical Operator4 : Logic  Operator=OR  AllPortsSameDT=off  OutDataTypeStr=boolean
  Relational Operator : RelationalOperator  Operator=<=  OutDataTypeStr=boolean  RndMeth=Simplest
  Relational Operator1 : RelationalOperator  Operator=<=  OutDataTypeStr=boolean  RndMeth=Simplest
  data1 : Lookup_n-D  NumberOfTableDimensions=1  BreakpointsForDimension1=[0,20,40,60,80,100,120,140]  Table=[1.5,1.5,1.45,1.45,1.4,1.4,1.4,1.4]  RndMeth=Simplest  InputSameDT=on
  data3 : Lookup_n-D  NumberOfTableDimensions=1  BreakpointsForDimension1=[0,40,45,55,60,65,70,95,115,140]  Table=[2.5,2.5,2.5,2.5,3,3,3,3,3.2,3.2]  RndMeth=Simplest  InputSameDT=on
  data4 : Lookup_n-D  NumberOfTableDimensions=1  BreakpointsForDimension1=[0,40,45,55,60,65,70,95,115,140]  Table=[1.4,1.5,1.7,1.7,2,2,2,2,2.5,2.5]  RndMeth=Simplest  InputSameDT=on
  TOS_ACC_DyConfirm : Outport
  wires:
  Object_DX/1 -> Bus Creator/2
  Object_DY/1 -> Bus Creator/1
  Relational Operator/1 -> Logical Operator/1
  Abs/1 -> data4/1
  data4/1 -> Relational Operator/2
  Abs1/1 -> Relational Operator/1
  <Object_Type>/1 -> Bus Creator/3
  Bus Selector/1 -> Data Type Conversion2/1  "<Object_Type>"
  Compare To Constant3/1 -> Logical Operator1/1
  Bus Selector2/1 -> Abs/1  "<Object_DX>"
  Bus Selector1/1 -> Abs1/1  "<Object_DY>"
  Data Type Conversion2/1 -> Compare To Constant7/1, Compare To Constant6/1, Compare To Constant5/1, Compare To Constant4/1, Compare To Constant2/1, Compare To Constant1/1, Compare To Constant3/1
  Compare To Constant1/1 -> Logical Operator1/2
  Compare To Constant2/1 -> Logical Operator1/3
  Compare To Constant4/1 -> Logical Operator1/4
  Compare To Constant5/1 -> Logical Operator1/5
  Compare To Constant6/1 -> Logical Operator1/6
  Compare To Constant7/1 -> Logical Operator1/7
  Logical Operator1/1 -> Logical Operator/2
  Logical Operator3/1 -> Logical Operator2/2
  Compare To Constant8/1 -> Logical Operator3/2
  Data Type Conversion1/1 -> Compare To Constant10/1, Compare To Constant8/1
  Bus Selector4/1 -> Abs3/1  "<Object_DY>"
  Bus Selector5/1 -> Abs2/1  "<Object_DX>"
  Compare To Constant10/1 -> Logical Operator3/1
  Bus Selector3/1 -> Data Type Conversion1/1  "<Object_Type>"
  Bus Creator/1 -> Bus Selector2/1, Bus Selector4/1, Bus Selector3/1, Bus Selector5/1, Bus Selector/1, Bus Selector1/1
  Abs3/1 -> Relational Operator1/1
  data3/1 -> Relational Operator1/2
  Abs2/1 -> data3/1
  Relational Operator1/1 -> Logical Operator2/1
  Logical Operator/1 -> Logical Operator4/1
  Logical Operator2/1 -> Logical Operator4/2
  Logical Operator4/1 -> TOS_ACC_DyConfirm/1

== system PubIfDecisionTOS_MDL/TOS_20201112/TOS_2012080320/TOS/ACC/TOS_ACCCurrentLane/ACC_CurrentLane_Target/TOS_ACC_P0/ACC_P0_Targe/ACC_P0_Targe/TOS_ACC_DyConfirm/TOS_ACC_DyConfirm_V3.15 ==
  Object_DY : Inport
  Object_DX : Inport  Port=2
  Object_Type : Inport  Port=3
  object_MovingState : Inport  Port=4
  Abs{,1..7} (8 alike) : Abs
  Bus Creator : BusCreator  Inputs=4
  Bus Selector1 : BusSelector  OutputSignals=Object_DY,Object_DX
  Bus Selector3 : BusSelector  OutputSignals=Object_DY,Object_DX,Object_Type
  Bus Selector6 : BusSelector  OutputSignals=Object_DY,Object_DX,object_MovingState
  Bus Selector7 : BusSelector  OutputSignals=Object_DY,Object_DX,Object_Type
  Compare To Constant1 : simulink/Logic and Bit Operations/Compare To Constant  relop===  const=OFM_OBJ_TYPE_E.UNKNOWN_TYPE  OutDataTypeStr=boolean
      settings: AttributesFormatString=OFM_OBJ_TYPE_E.UNKNOWN_TYPE = 1
  Compare To Constant10 : simulink/Logic and Bit Operations/Compare To Constant  relop===  const=OFM_OBJ_TYPE_E.CAR  OutDataTypeStr=boolean
      settings: AttributesFormatString=OFM_OBJ_TYPE_E.CAR = 2
  Compare To Constant11 : simulink/Logic and Bit Operations/Compare To Constant  relop===  const=OFM_OBJ_MOVINGSTATE_E.STATIONARY  OutDataTypeStr=boolean
      settings: AttributesFormatString=OFM_OBJ_MOVINGSTATE_E.UNKNOWN = 3
  Compare To Constant2 : simulink/Logic and Bit Operations/Compare To Constant  relop===  const=OFM_OBJ_TYPE_E.MOTORBIKE  OutDataTypeStr=boolean
      settings: AttributesFormatString=OFM_OBJ_TYPE_E.MOTORBIKE = 4
  Compare To Constant3 : simulink/Logic and Bit Operations/Compare To Constant  relop===  const=OFM_OBJ_TYPE_E.PEDESTRIAN  OutDataTypeStr=boolean
      settings: AttributesFormatString=OFM_OBJ_TYPE_E.PEDESTRIAN = 6
  Compare To Constant4 : simulink/Logic and Bit Operations/Compare To Constant  relop===  const=OFM_OBJ_TYPE_E.BICYCLE  OutDataTypeStr=boolean
      settings: AttributesFormatString=OFM_OBJ_TYPE_E.BICYCLE = 5
  Compare To Constant5 : simulink/Logic and Bit Operations/Compare To Constant  relop===  const=OFM_OBJ_TYPE_E.GENERAL_OBJECT  OutDataTypeStr=boolean
      settings: AttributesFormatString=OFM_OBJ_TYPE_E.GENERAL_OBJECT = 7
  Compare To Constant6 : simulink/Logic and Bit Operations/Compare To Constant  relop===  const=OFM_OBJ_TYPE_E.ANIMAL  OutDataTypeStr=boolean
      settings: AttributesFormatString=OFM_OBJ_TYPE_E.ANIMAL = 8
  Compare To Constant8 : simulink/Logic and Bit Operations/Compare To Constant  relop===  const=OFM_OBJ_TYPE_E.TRUCK  OutDataTypeStr=boolean
      settings: AttributesFormatString=OFM_OBJ_TYPE_E.TRUCK = 3
  Compare To Constant9 : simulink/Logic and Bit Operations/Compare To Constant  relop===  const=OFM_OBJ_MOVINGSTATE_E.UNKNOWN  OutDataTypeStr=boolean
      settings: AttributesFormatString=OFM_OBJ_MOVINGSTATE_E.UNKNOWN = 1
  Data Type Conversion1 : DataTypeConversion  OutDataTypeStr=Enum: OFM_OBJ_TYPE_E
  Data Type Conversion2 : DataTypeConversion  OutDataTypeStr=Enum: OFM_OBJ_TYPE_E
  Data Type Conversion3 : DataTypeConversion  OutDataTypeStr=Enum: OFM_OBJ_MOVINGSTATE_E
  Logical Operator1 : Logic  Operator=OR  Inputs=6  AllPortsSameDT=off  OutDataTypeStr=boolean
  Logical Operator3 : Logic  Operator=OR  AllPortsSameDT=off  OutDataTypeStr=boolean
  Logical Operator6 : Logic  Operator=OR  AllPortsSameDT=off  OutDataTypeStr=boolean
  Relational Operator{,1..3} (4 alike) : RelationalOperator  Operator=<=  OutDataTypeStr=boolean  RndMeth=Simplest
  Switch : Switch  Criteria=u2 > Threshold
  Switch1 : Switch  Criteria=u2 > Threshold
  Switch2 : Switch  Criteria=u2 > Threshold
  data1 : Lookup_n-D  NumberOfTableDimensions=1  BreakpointsForDimension1=[0,20,40,60,80,100,120,140]  Table=[1.5,1.5,1.45,1.45,1.4,1.4,1.4,1.4]  RndMeth=Simplest  InputSameDT=on
  data3 : Lookup_n-D  NumberOfTableDimensions=1  BreakpointsForDimension1=[0,20,40,60,80,100,120,140]  Table=[1.4,1.4,1.3,1.3,1.2,1.2,1.2,1.2]  RndMeth=Simplest  InputSameDT=on
  data4 : Lookup_n-D  NumberOfTableDimensions=1  BreakpointsForDimension1=[0,20,40,60,80,100,120,140]  Table=[1.4,1.4,1.3,1.3,1.2,1.2,1.2,1.2]  RndMeth=Simplest  InputSameDT=on
  data5 : Lookup_n-D  NumberOfTableDimensions=1  BreakpointsForDimension1=[0,20,40,60,80,100,120,140]  Table=[1.9,1.9,1.85,1.85,1.8,1.8,1.8,1.8]  RndMeth=Simplest  InputSameDT=on
  TOS_ACC_DyConfirm : Outport
  TOS_ACC_P0_P1_DyConfirm_1_ObserVale : Outport  Port=2
  TOS_ACC_P0_P1_DyConfirm_2_ObserVale : Outport  Port=3
  TOS_ACC_P0_P1_DyConfirm_3_ObserVale : Outport  Port=4
  wires:
  Switch/1 -> TOS_ACC_DyConfirm/1
  Abs2/1 -> data5/1
  data5/1 -> Relational Operator1/2
  Abs3/1 -> Relational Operator1/1
  Bus Selector7/3 -> Data Type Conversion1/1  "<Object_Type>"
  Compare To Constant10/1 -> Logical Operator3/1
  Bus Selector7/2 -> Abs2/1  "<Object_DX>"
  Bus Selector7/1 -> Abs3/1  "<Object_DY>"
  Data Type Conversion1/1 -> Compare To Constant8/1, Compare To Constant10/1
  Compare To Constant8/1 -> Logical Operator3/2
  Logical Operator1/1 -> [TOS_ACC_P0_P1_DyConfirm_3_ObserVale], Switch2/2
  Compare To Constant6/1 -> Logical Operator1/6
  Compare To Constant5/1 -> Logical Operator1/5
  Compare To Constant4/1 -> Logical Operator1/4
  Compare To Constant2/1 -> Logical Operator1/3
  Compare To Constant1/1 -> Logical Operator1/2
  Data Type Conversion2/1 -> Compare To Constant3/1, Compare To Constant6/1, Compare To Constant5/1, Compare To Constant4/1, Compare To Constant2/1, Compare To Constant1/1
  Bus Selector3/1 -> Abs1/1  "<Object_DY>"
  Bus Selector3/2 -> Abs/1  "<Object_DX>"
  Compare To Constant3/1 -> Logical Operator1/1
  Bus Selector3/3 -> Data Type Conversion2/1  "<Object_Type>"
  Object_Type/1 -> Bus Creator/3  "Object_Type"
  Abs1/1 -> Relational Operator/1
  data3/1 -> Relational Operator/2
  Abs/1 -> data3/1
  Relational Operator/1 -> Switch2/1
  Object_DY/1 -> Bus Creator/1  "Object_DY"
  Object_DX/1 -> Bus Creator/2  "Object_DX"
  Bus Creator/1 -> Bus Selector1/1, Bus Selector3/1, Bus Selector7/1, Bus Selector6/1
  Compare To Constant11/1 -> Logical Operator6/2
  Compare To Constant9/1 -> Logical Operator6/1
  object_MovingState/1 -> Bus Creator/4  "object_MovingState"
  Bus Selector6/3 -> Data Type Conversion3/1  "<object_MovingState>"
  Bus Selector6/1 -> Abs4/1  "<Object_DY>"
  Bus Selector6/2 -> Abs5/1  "<Object_DX>"
  Abs5/1 -> data1/1
  data1/1 -> Relational Operator2/2
  Abs4/1 -> Relational Operator2/1
  Logical Operator6/1 -> [TOS_ACC_P0_P1_DyConfirm_1_ObserVale], Switch/2
  Relational Operator2/1 -> Switch/1
  Logical Operator3/1 -> [TOS_ACC_P0_P1_DyConfirm_2_ObserVale], Switch1/2
  Relational Operator1/1 -> Switch1/1
  Switch1/1 -> Switch/3
  Switch2/1 -> Switch1/3
  Bus Selector1/2 -> Abs6/1  "<Object_DX>"
  Bus Selector1/1 -> Abs7/1  "<Object_DY>"
  Abs6/1 -> data4/1
  data4/1 -> Relational Operator3/2
  Abs7/1 -> Relational Operator3/1
  Relational Operator3/1 -> Switch2/3
  [TOS_ACC_P0_P1_DyConfirm_1_ObserVale] -> TOS_ACC_P0_P1_DyConfirm_1_ObserVale/1
  [TOS_ACC_P0_P1_DyConfirm_2_ObserVale] -> TOS_ACC_P0_P1_DyConfirm_2_ObserVale/1
  [TOS_ACC_P0_P1_DyConfirm_3_ObserVale] -> TOS_ACC_P0_P1_DyConfirm_3_ObserVale/1
  Data Type Conversion3/1 -> Compare To Constant11/1, Compare To Constant9/1  "object_MovingState"

== system PubIfDecisionTOS_MDL/TOS_20201112/TOS_2012080320/TOS/ACC/TOS_ACCCurrentLane/ACC_CurrentLane_Target/TOS_ACC_P0/ACC_P0_Targe/ACC_P0_Targe/TOS_ACC_FusionTypeConfirm/Subsystem1 ==
  ObjMovState : Inport
  ACC_Target_ID_K1 : Inport  Port=2
  ACC_Target_ID_K2 : Inport  Port=3
  ACC_Target_MovState_K1 : Inport  Port=4
  ACC_Target_MovState_K2 : Inport  Port=5
  ObjectID : Inport  Port=6
  TOS_ObjMovStateCfmFlow1 : Stateflow chart  TreatAsAtomicUnit=on
  TOS_ObjMovStateCfm : Outport
  wires:
  TOS_ObjMovStateCfmFlow1/1(TOS_ObjMovStateCfm) -> TOS_ObjMovStateCfm/1
  ACC_Target_ID_K1/1 -> TOS_ObjMovStateCfmFlow1/1(Target_ID_K1)
  ACC_Target_ID_K2/1 -> TOS_ObjMovStateCfmFlow1/2(Target_ID_K2)
  ACC_Target_MovState_K1/1 -> TOS_ObjMovStateCfmFlow1/3(Target_MovState_K1)
  ACC_Target_MovState_K2/1 -> TOS_ObjMovStateCfmFlow1/4(Target_MovState_K2)
  ObjMovState/1 -> TOS_ObjMovStateCfmFlow1/5(ObjMovState)
  ObjectID/1 -> TOS_ObjMovStateCfmFlow1/6(ObjectID)

== system PubIfDecisionTOS_MDL/TOS_20201112/TOS_2012080320/TOS/ACC/TOS_ACCCurrentLane/ACC_CurrentLane_Target/TOS_ACC_P0/ACC_P0_Targe/ACC_P0_Targe/TOS_ACC_FusionTypeConfirm/TOS_ACCFusionTypeAborDly ==
  ACC_TargetP0_ID_K1 : Inport
  ObjectID : Inport  Port=2
  TOS_ACCFusionType : Inport  Port=3
  If : If  IfExpression=u1
  If Action Subsystem : Subsystem  TreatAsAtomicUnit=on
  If Action Subsystem1 : Subsystem  TreatAsAtomicUnit=on
  Merge : Merge
  Relational Operator : RelationalOperator  Operator===  OutDataTypeStr=boolean  RndMeth=Simplest
  TOS_ACCFusionTypeFilt : Outport
  wires:
  If/1 -> If Action Subsystem1/Action
  TOS_ACCFusionType/1 -> If Action Subsystem1/1(TOS_ACCFusionType), If Action Subsystem/1(TOS_ACCFusionType)
  If/2 -> If Action Subsystem/Action
  ACC_TargetP0_ID_K1/1 -> Relational Operator/1
  ObjectID/1 -> Relational Operator/2
  Relational Operator/1 -> If/1
  If Action Subsystem1/1(TOS_ACCFusionTypeFilt) -> Merge/1
  If Action Subsystem/1(TOS_ACCFusionTypeFilt) -> Merge/2
  Merge/1 -> TOS_ACCFusionTypeFilt/1

== system PubIfDecisionTOS_MDL/TOS_20201112/TOS_2012080320/TOS/ACC/TOS_ACCCurrentLane/ACC_CurrentLane_Target/TOS_ACC_P0/ACC_P0_Targe/ACC_P0_Targe/TOS_ACC_ObjTypeConfirm/Subsystem ==
  ObjMovState : Inport
  ACC_Target_ID_K1 : Inport  Port=2
  ACC_Target_ID_K2 : Inport  Port=3
  ACC_Target_MovState_K1 : Inport  Port=4
  ACC_Target_MovState_K2 : Inport  Port=5
  ObjectID : Inport  Port=6
  TOS_ObjMovStateCfmFlow1 : Stateflow chart  TreatAsAtomicUnit=on
  TOS_ObjMovStateCfm : Outport
  wires:
  TOS_ObjMovStateCfmFlow1/1(TOS_ObjMovStateCfm) -> TOS_ObjMovStateCfm/1
  ACC_Target_ID_K1/1 -> TOS_ObjMovStateCfmFlow1/1(ACC_TargetP0_ID_K1)
  ACC_Target_ID_K2/1 -> TOS_ObjMovStateCfmFlow1/2(ACC_TargetP0_ID_K2)
  ACC_Target_MovState_K1/1 -> TOS_ObjMovStateCfmFlow1/3(ACC_TargetP0_MovState_K1)
  ACC_Target_MovState_K2/1 -> TOS_ObjMovStateCfmFlow1/4(ACC_TargetP0_MovState_K2)
  ObjMovState/1 -> TOS_ObjMovStateCfmFlow1/5(ObjMovState)
  ObjectID/1 -> TOS_ObjMovStateCfmFlow1/6(ObjectID)

== system PubIfDecisionTOS_MDL/TOS_20201112/TOS_2012080320/TOS/ACC/TOS_ACCCurrentLane/ACC_CurrentLane_Target/TOS_ACC_P0/ACC_P0_Targe/ACC_P0_Targe/TOS_ACC_ObjTypeConfirm/TOS_ACCObjTypeAborDly ==
  ACC_Target_ID_K1 : Inport
  ObjectID : Inport  Port=2
  TOS_ACCObjType : Inport  Port=3
  If : If  IfExpression=u1
  If Action Subsystem : Subsystem  TreatAsAtomicUnit=on
  If Action Subsystem1 : Subsystem  TreatAsAtomicUnit=on
  Merge : Merge
  Relational Operator : RelationalOperator  Operator===  OutDataTypeStr=boolean  RndMeth=Simplest
  TOS_ACCObjTypeFilt : Outport
  wires:
  If/1 -> If Action Subsystem1/Action
  TOS_ACCObjType/1 -> If Action Subsystem1/1(TOS_ACCFusionType), If Action Subsystem/1(TOS_ACCFusionType)
  If/2 -> If Action Subsystem/Action
  ACC_Target_ID_K1/1 -> Relational Operator/1
  ObjectID/1 -> Relational Operator/2
  Relational Operator/1 -> If/1
  If Action Subsystem1/1(TOS_ACCFusionTypeFilt) -> Merge/1
  If Action Subsystem/1(TOS_ACCFusionTypeFilt) -> Merge/2
  Merge/1 -> TOS_ACCObjTypeFilt/1
